simulink model "task_A_mod"  (R2013b)
settings: Solver=ode45  StartTime=0.0  StopTime=10.0  RelTol=1e-3
values from neighbouring files (symbols this model uses):
  A = [0,1;-c/m,-beta/m]    [task_A_scr.m]    (also in task_B_scr.m = A*(16*lamda/(c*ro*h^2)); task_C1_scr.m = A*(16*lamda/(c*ro*h^2)); task_C_scr.m = A*(16*lamda/(c*ro*h^2)); task_D1_scr.m = A*(16*lamda/(c*ro*h^2)))
  B = [0;1]    [task_A_scr.m]    (also in task_B_scr.m = B*(4/(c*ro*h)); task_C1_scr.m = B*(4/(c*ro*h)); task_C_scr.m = B*(4/(c*ro*h)); task_D1_scr.m = B*(4/(c*ro*h)))
settings Model: Creator=Yurii  LastModifiedBy=Yurii

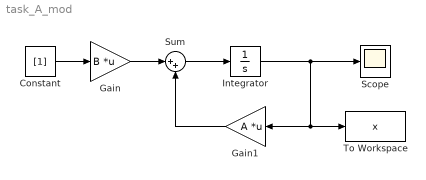
== system task_A_mod ==
  Constant : Constant  Value=[1]
  Gain : Gain  Gain=B  Multiplication=Matrix(K*u)
  Gain1 : Gain  Gain=A  Multiplication=Matrix(K*u)
  Integrator : Integrator
  Scope : Scope
  Sum : Sum  Inputs=|++
  To Workspace : ToWorkspace  VariableName=x  SampleTime=-1  SaveFormat=Timeseries
  wires:
  Constant/1 -> Gain/1
  Gain/1 -> Sum/1
  Sum/1 -> Integrator/1
  Gain1/1 -> Sum/2
  Integrator/1 -> Gain1/1, To Workspace/1, Scope/1
